simulink model "Backhoe_TiltCyl_PIopt"  (R2018a)
settings: Solver=ode23t  StartTime=0.0  StopTime=30  MaxStep=0.01  RelTol=1e-3  EnableMultiTasking=on
PreLoadFcn:
  | Kp_Final = 19.24;
  | Ki_Final = 0.5024;
  | 
  | Kp_Init = 0.1;
  | Ki_Init = 0.02;
  | 
  | 
  | Kp = Kp_Init;
  | Ki = Ki_Init;
PostLoadFcn:
  | warning off Simulink:Engine:UsingDefaultMaxStepSize
  | warning off Simulink:blocks:MatchingFromNotFound
  | warning off Simulink:Engine:SaveWithParameterizedLinks_Warning
  | warning off Simulink:Engine:SolverMinStepSizeWarnForDAE
model workspace (MAT data in the model file):
  Backhoe_TiltCyl_sdosession = sldodialogs.data.SessionData
  Backhoe_TiltCyl_sdosession.Version = '3.0'
  Backhoe_TiltCyl_sdosession.Data.ModelName = 'Backhoe_TiltCyl_v2'
  Backhoe_TiltCyl_sdosession.Data.GUIOptions.NoPromptClose = 0
  Backhoe_TiltCyl_sdosession.Data.ToolData.PlotManager.Plots.Class = 'sldoplots.TimePlot'
  Backhoe_TiltCyl_sdosession.Data.ToolData.PlotManager.Plots.Sources = {'Bucket_Angle'}
  Backhoe_TiltCyl_sdosession.Data.ToolData.ResponseOptimization.DesignVariables = 'DesignVars'
  Backhoe_TiltCyl_sdosession.Data.ToolData.ResponseOptimization.UncertainVariables = ''
  Backhoe_TiltCyl_sdosession.Data.ToolData.ResponseOptimization.Options = sdo.OptimizeOptions
  Backhoe_TiltCyl_sdosession.Data.ToolData.ResponseOptimization.Options.MethodOptions.Display = 'iter'
  Backhoe_TiltCyl_sdosession.Data.ToolData.ResponseOptimization.Options.MethodOptions.MaxFunEvals = Inf
  Backhoe_TiltCyl_sdosession.Data.ToolData.ResponseOptimization.Options.MethodOptions.MaxIter = 100
  Backhoe_TiltCyl_sdosession.Data.ToolData.ResponseOptimization.Options.MethodOptions.TolFun = 0.001
  Backhoe_TiltCyl_sdosession.Data.ToolData.ResponseOptimization.Options.MethodOptions.TolX = 0.001
  Backhoe_TiltCyl_sdosession.Data.ToolData.ResponseOptimization.Options.MethodOptions.FunValCheck = 'off'
  Backhoe_TiltCyl_sdosession.Data.ToolData.ResponseOptimization.Options.MethodOptions.OutputFcn = []
  Backhoe_TiltCyl_sdosession.Data.ToolData.ResponseOptimization.Options.MethodOptions.PlotFcns = []
  Backhoe_TiltCyl_sdosession.Data.ToolData.ResponseOptimization.Options.MethodOptions.ActiveConstrTol = []
  Backhoe_TiltCyl_sdosession.Data.ToolData.ResponseOptimization.Options.MethodOptions.Algorithm = 'active-set'
  Backhoe_TiltCyl_sdosession.Data.ToolData.ResponseOptimization.Options.MethodOptions.AlwaysHonorConstraints = 'bounds'
  Backhoe_TiltCyl_sdosession.Data.ToolData.ResponseOptimization.Options.MethodOptions.BranchStrategy = []
  Backhoe_TiltCyl_sdosession.Data.ToolData.ResponseOptimization.Options.MethodOptions.DerivativeCheck = 'off'
  Backhoe_TiltCyl_sdosession.Data.ToolData.ResponseOptimization.Options.MethodOptions.Diagnostics = 'off'
  Backhoe_TiltCyl_sdosession.Data.ToolData.ResponseOptimization.Options.MethodOptions.DiffMaxChange = Inf
  Backhoe_TiltCyl_sdosession.Data.ToolData.ResponseOptimization.Options.MethodOptions.DiffMinChange = 0
  Backhoe_TiltCyl_sdosession.Data.ToolData.ResponseOptimization.Options.MethodOptions.FinDiffRelStep = []
  Backhoe_TiltCyl_sdosession.Data.ToolData.ResponseOptimization.Options.MethodOptions.FinDiffType = 'forward'
  Backhoe_TiltCyl_sdosession.Data.ToolData.ResponseOptimization.Options.MethodOptions.GoalsExactAchieve = []
  Backhoe_TiltCyl_sdosession.Data.ToolData.ResponseOptimization.Options.MethodOptions.GradConstr = 'on'
  Backhoe_TiltCyl_sdosession.Data.ToolData.ResponseOptimization.Options.MethodOptions.GradObj = 'on'
  Backhoe_TiltCyl_sdosession.Data.ToolData.ResponseOptimization.Options.MethodOptions.HessFcn = []
  Backhoe_TiltCyl_sdosession.Data.ToolData.ResponseOptimization.Options.MethodOptions.Hessian = []
  Backhoe_TiltCyl_sdosession.Data.ToolData.ResponseOptimization.Options.MethodOptions.HessMult = []
  Backhoe_TiltCyl_sdosession.Data.ToolData.ResponseOptimization.Options.MethodOptions.HessPattern = 'sparse(ones(numberofvariables))'
  Backhoe_TiltCyl_sdosession.Data.ToolData.ResponseOptimization.Options.MethodOptions.HessUpdate = []
  Backhoe_TiltCyl_sdosession.Data.ToolData.ResponseOptimization.Options.MethodOptions.InitialHessType = []
  Backhoe_TiltCyl_sdosession.Data.ToolData.ResponseOptimization.Options.MethodOptions.InitialHessMatrix = []
  Backhoe_TiltCyl_sdosession.Data.ToolData.ResponseOptimization.Options.MethodOptions.InitBarrierParam = 0.1
  Backhoe_TiltCyl_sdosession.Data.ToolData.ResponseOptimization.Options.MethodOptions.InitTrustRegionRadius = 'sqrt(numberofvariables)'
  Backhoe_TiltCyl_sdosession.Data.ToolData.ResponseOptimization.Options.MethodOptions.Jacobian = []
  Backhoe_TiltCyl_sdosession.Data.ToolData.ResponseOptimization.Options.MethodOptions.JacobMult = []
  Backhoe_TiltCyl_sdosession.Data.ToolData.ResponseOptimization.Options.MethodOptions.JacobPattern = []
  Backhoe_TiltCyl_sdosession.Data.ToolData.ResponseOptimization.Options.MethodOptions.LargeScale = 'on'
  Backhoe_TiltCyl_sdosession.Data.ToolData.ResponseOptimization.Options.MethodOptions.LineSearchType = []
  Backhoe_TiltCyl_sdosession.Data.ToolData.ResponseOptimization.Options.MethodOptions.MaxNodes = []
  Backhoe_TiltCyl_sdosession.Data.ToolData.ResponseOptimization.Options.MethodOptions.MaxPCGIter = 'max(1,floor(numberofvariables/2))'
  Backhoe_TiltCyl_sdosession.Data.ToolData.ResponseOptimization.Options.MethodOptions.MaxProjCGIter = '2*(numberofvariables-numberofequalities)'
  Backhoe_TiltCyl_sdosession.Data.ToolData.ResponseOptimization.Options.MethodOptions.MaxRLPIter = []
  Backhoe_TiltCyl_sdosession.Data.ToolData.ResponseOptimization.Options.MethodOptions.MaxSQPIter = '10*max(numberofvariables,numberofinequalities+numberofbounds)'
  Backhoe_TiltCyl_sdosession.Data.ToolData.ResponseOptimization.Options.MethodOptions.MaxTime = []
  Backhoe_TiltCyl_sdosession.Data.ToolData.ResponseOptimization.Options.MethodOptions.MeritFunction = []
  Backhoe_TiltCyl_sdosession.Data.ToolData.ResponseOptimization.Options.MethodOptions.MinAbsMax = []
  Backhoe_TiltCyl_sdosession.Data.ToolData.ResponseOptimization.Options.MethodOptions.NodeDisplayInterval = []
  Backhoe_TiltCyl_sdosession.Data.ToolData.ResponseOptimization.Options.MethodOptions.NodeSearchStrategy = []
  Backhoe_TiltCyl_sdosession.Data.ToolData.ResponseOptimization.Options.MethodOptions.NoStopIfFlatInfeas = 'on'
  Backhoe_TiltCyl_sdosession.Data.ToolData.ResponseOptimization.Options.MethodOptions.ObjectiveLimit = -1e+20
  Backhoe_TiltCyl_sdosession.Data.ToolData.ResponseOptimization.Options.MethodOptions.PhaseOneTotalScaling = 'on'
  Backhoe_TiltCyl_sdosession.Data.ToolData.ResponseOptimization.Options.MethodOptions.Preconditioner = []
  Backhoe_TiltCyl_sdosession.Data.ToolData.ResponseOptimization.Options.MethodOptions.PrecondBandWidth = Inf
  Backhoe_TiltCyl_sdosession.Data.ToolData.ResponseOptimization.Options.MethodOptions.RelLineSrchBnd = 9
  Backhoe_TiltCyl_sdosession.Data.ToolData.ResponseOptimization.Options.MethodOptions.RelLineSrchBndDuration = Inf
  Backhoe_TiltCyl_sdosession.Data.ToolData.ResponseOptimization.Options.MethodOptions.ScaleProblem = 'none'
  Backhoe_TiltCyl_sdosession.Data.ToolData.ResponseOptimization.Options.MethodOptions.Simplex = []
  Backhoe_TiltCyl_sdosession.Data.ToolData.ResponseOptimization.Options.MethodOptions.SubproblemAlgorithm = 'ldl-factorization'
  Backhoe_TiltCyl_sdosession.Data.ToolData.ResponseOptimization.Options.MethodOptions.TolCon = 0.001
  Backhoe_TiltCyl_sdosession.Data.ToolData.ResponseOptimization.Options.MethodOptions.TolConSQP = 1e-06
  Backhoe_TiltCyl_sdosession.Data.ToolData.ResponseOptimization.Options.MethodOptions.TolGradCon = 1e-06
  Backhoe_TiltCyl_sdosession.Data.ToolData.ResponseOptimization.Options.MethodOptions.TolPCG = 0.1
  Backhoe_TiltCyl_sdosession.Data.ToolData.ResponseOptimization.Options.MethodOptions.TolProjCG = 0.01
  Backhoe_TiltCyl_sdosession.Data.ToolData.ResponseOptimization.Options.MethodOptions.TolProjCGAbs = 1e-10
  Backhoe_TiltCyl_sdosession.Data.ToolData.ResponseOptimization.Options.MethodOptions.TolRLPFun = []
  Backhoe_TiltCyl_sdosession.Data.ToolData.ResponseOptimization.Options.MethodOptions.TolXInteger = []
  Backhoe_TiltCyl_sdosession.Data.ToolData.ResponseOptimization.Options.MethodOptions.TypicalX = 'ones(numberofvariables,1)'
  Backhoe_TiltCyl_sdosession.Data.ToolData.ResponseOptimization.Options.MethodOptions.UseParallel = 'never'
  Backhoe_TiltCyl_sdosession.Data.ToolData.ResponseOptimization.Options.OptimizedModel = 'Backhoe_TiltCyl_v2'
  Backhoe_TiltCyl_sdosession.Data.ToolData.ResponseOptimization.GUIOptions.ShowProgress = 1
  Backhoe_TiltCyl_sdosession.Data.ToolData.ResponseOptimization.GUIOptions.UpdatePlots = 1
  Backhoe_TiltCyl_sdosession.Data.ToolData.ResponseOptimization.GUIOptions.UpdateModel = 1
  Backhoe_TiltCyl_sdosession.Data.ToolData.ResponseOptimization.GUIOptions.UpdateDesign = 'overwrite'
  Backhoe_TiltCyl_sdosession.Data.ToolData.ResponseOptimization.GUIOptions.SaveReport = 0
  Backhoe_TiltCyl_sdosession.Data.ToolData.ResponseOptimization.GUIOptions.SaveRequirementValue = 1
  Backhoe_TiltCyl_sdosession.Data.ToolData.ResponseOptimization.DataToPlot = ''
  Backhoe_TiltCyl_sdosession.Data.ToolData.ResponseOptimization.LinOptions = linearize.OldLinoptions
  Backhoe_TiltCyl_sdosession.Data.ToolData.ResponseOptimization.LinOptions.OptimizerType = 'graddescent-elim'
  Backhoe_TiltCyl_sdosession.Data.ToolData.ResponseOptimization.LinOptions.OptimizationOptions.Algorithm = 'active-set'
  Backhoe_TiltCyl_sdosession.Data.ToolData.ResponseOptimization.LinOptions.OptimizationOptions.AlwaysHonorConstraints = 'bounds'
  Backhoe_TiltCyl_sdosession.Data.ToolData.ResponseOptimization.LinOptions.OptimizationOptions.DerivativeCheck = 'off'
  Backhoe_TiltCyl_sdosession.Data.ToolData.ResponseOptimization.LinOptions.OptimizationOptions.Diagnostics = 'off'
  Backhoe_TiltCyl_sdosession.Data.ToolData.ResponseOptimization.LinOptions.OptimizationOptions.DiffMaxChange = Inf
  Backhoe_TiltCyl_sdosession.Data.ToolData.ResponseOptimization.LinOptions.OptimizationOptions.DiffMinChange = 0
  Backhoe_TiltCyl_sdosession.Data.ToolData.ResponseOptimization.LinOptions.OptimizationOptions.Display = 'off'
  Backhoe_TiltCyl_sdosession.Data.ToolData.ResponseOptimization.LinOptions.OptimizationOptions.FinDiffRelStep = []
  Backhoe_TiltCyl_sdosession.Data.ToolData.ResponseOptimization.LinOptions.OptimizationOptions.FinDiffType = 'forward'
  Backhoe_TiltCyl_sdosession.Data.ToolData.ResponseOptimization.LinOptions.OptimizationOptions.FunValCheck = 'off'
  Backhoe_TiltCyl_sdosession.Data.ToolData.ResponseOptimization.LinOptions.OptimizationOptions.GradConstr = 'off'
  Backhoe_TiltCyl_sdosession.Data.ToolData.ResponseOptimization.LinOptions.OptimizationOptions.GradObj = 'off'
  Backhoe_TiltCyl_sdosession.Data.ToolData.ResponseOptimization.LinOptions.OptimizationOptions.HessFcn = []
  Backhoe_TiltCyl_sdosession.Data.ToolData.ResponseOptimization.LinOptions.OptimizationOptions.Hessian = []
  Backhoe_TiltCyl_sdosession.Data.ToolData.ResponseOptimization.LinOptions.OptimizationOptions.HessMult = []
  Backhoe_TiltCyl_sdosession.Data.ToolData.ResponseOptimization.LinOptions.OptimizationOptions.HessPattern = 'sparse(ones(numberOfVariables))'
  Backhoe_TiltCyl_sdosession.Data.ToolData.ResponseOptimization.LinOptions.OptimizationOptions.InitBarrierParam = 0.1
  Backhoe_TiltCyl_sdosession.Data.ToolData.ResponseOptimization.LinOptions.OptimizationOptions.InitTrustRegionRadius = 'sqrt(numberOfVariables)'
  Backhoe_TiltCyl_sdosession.Data.ToolData.ResponseOptimization.LinOptions.OptimizationOptions.MaxFunEvals = 600
  Backhoe_TiltCyl_sdosession.Data.ToolData.ResponseOptimization.LinOptions.OptimizationOptions.MaxIter = 400
  Backhoe_TiltCyl_sdosession.Data.ToolData.ResponseOptimization.LinOptions.OptimizationOptions.MaxPCGIter = 'max(1,floor(numberOfVariables/2))'
  Backhoe_TiltCyl_sdosession.Data.ToolData.ResponseOptimization.LinOptions.OptimizationOptions.MaxProjCGIter = '2*(numberOfVariables-numberOfEqualities)'
  Backhoe_TiltCyl_sdosession.Data.ToolData.ResponseOptimization.LinOptions.OptimizationOptions.MaxSQPIter = '10*max(numberOfVariables,numberOfInequalities+numberOfBounds)'
  Backhoe_TiltCyl_sdosession.Data.ToolData.ResponseOptimization.LinOptions.OptimizationOptions.ObjectiveLimit = -1e+20
  Backhoe_TiltCyl_sdosession.Data.ToolData.ResponseOptimization.LinOptions.OptimizationOptions.OutputFcn = []
  Backhoe_TiltCyl_sdosession.Data.ToolData.ResponseOptimization.LinOptions.OptimizationOptions.PlotFcns = []
  Backhoe_TiltCyl_sdosession.Data.ToolData.ResponseOptimization.LinOptions.OptimizationOptions.PrecondBandWidth = 0
  Backhoe_TiltCyl_sdosession.Data.ToolData.ResponseOptimization.LinOptions.OptimizationOptions.RelLineSrchBnd = []
  Backhoe_TiltCyl_sdosession.Data.ToolData.ResponseOptimization.LinOptions.OptimizationOptions.RelLineSrchBndDuration = 1
  Backhoe_TiltCyl_sdosession.Data.ToolData.ResponseOptimization.LinOptions.OptimizationOptions.ScaleProblem = 'none'
  Backhoe_TiltCyl_sdosession.Data.ToolData.ResponseOptimization.LinOptions.OptimizationOptions.SubproblemAlgorithm = 'ldl-factorization'
  Backhoe_TiltCyl_sdosession.Data.ToolData.ResponseOptimization.LinOptions.OptimizationOptions.TolCon = 1e-06
  Backhoe_TiltCyl_sdosession.Data.ToolData.ResponseOptimization.LinOptions.OptimizationOptions.TolConSQP = 1e-06
  Backhoe_TiltCyl_sdosession.Data.ToolData.ResponseOptimization.LinOptions.OptimizationOptions.TolFun = 1e-06
  Backhoe_TiltCyl_sdosession.Data.ToolData.ResponseOptimization.LinOptions.OptimizationOptions.TolPCG = 0.1
  Backhoe_TiltCyl_sdosession.Data.ToolData.ResponseOptimization.LinOptions.OptimizationOptions.TolProjCG = 0.01
  Backhoe_TiltCyl_sdosession.Data.ToolData.ResponseOptimization.LinOptions.OptimizationOptions.TolProjCGAbs = 1e-10
  Backhoe_TiltCyl_sdosession.Data.ToolData.ResponseOptimization.LinOptions.OptimizationOptions.TolX = 1e-06
  Backhoe_TiltCyl_sdosession.Data.ToolData.ResponseOptimization.LinOptions.OptimizationOptions.TypicalX = 'ones(numberOfVariables,1)'
  Backhoe_TiltCyl_sdosession.Data.ToolData.ResponseOptimization.LinOptions.OptimizationOptions.UseParallel = 0
  Backhoe_TiltCyl_sdosession.Data.ToolData.ResponseOptimization.LinOptions.OptimizationOptions.Jacobian = 'off'
  Backhoe_TiltCyl_sdosession.Data.ToolData.ResponseOptimization.LinOptions.OptimizationOptions.LargeScale = 'off'
  Backhoe_TiltCyl_sdosession.Data.ToolData.ResponseOptimization.LocalRequirements.Requirement = 'SignalTracking'
  Backhoe_TiltCyl_sdosession.Data.ToolData.ResponseOptimization.LocalRequirements.Source = {'Bucket_Angle'}
  Backhoe_TiltCyl_sdosession.Data.ToolData.ResponseOptimization.LocalRequirements.Selected = 1
  Backhoe_TiltCyl_sdosession.Data.ToolData.ResponseOptimization.BlockRequirements = struct([])
  Backhoe_TiltCyl_sdosession.Data.OpenTabs = {'tabResponseOptimization'}
  Backhoe_TiltCyl_sdosession.Data.ToolType = 'ResponseOptimization'
  Backhoe_TiltCyl_sdosession.Data.Workspace.LocalWorkspace.Bucket_Angle = Simulink.SimulationData.Signal
  Backhoe_TiltCyl_sdosession.Data.Workspace.LocalWorkspace.Bucket_Angle.PortType = 'outport'
  Backhoe_TiltCyl_sdosession.Data.Workspace.LocalWorkspace.Bucket_Angle.BlockPath = Simulink.SimulationData.BlockPath
  Backhoe_TiltCyl_sdosession.Data.Workspace.LocalWorkspace.Bucket_Angle.BlockPath.path = {'Backhoe_TiltCyl_v2/Tilt Actuator'}
  Backhoe_TiltCyl_sdosession.Data.Workspace.LocalWorkspace.DesignVars(1) = param.Continuous
  Backhoe_TiltCyl_sdosession.Data.Workspace.LocalWorkspace.DesignVars(1).Minimum_ = 0
  Backhoe_TiltCyl_sdosession.Data.Workspace.LocalWorkspace.DesignVars(1).Scale_ = 0.25
  Backhoe_TiltCyl_sdosession.Data.Workspace.LocalWorkspace.DesignVars(1).Size_ = [1 1]
  Backhoe_TiltCyl_sdosession.Data.Workspace.LocalWorkspace.DesignVars(1).Value_ = 0.2
  Backhoe_TiltCyl_sdosession.Data.Workspace.LocalWorkspace.DesignVars(1).pID = paramid.Variable
  Backhoe_TiltCyl_sdosession.Data.Workspace.LocalWorkspace.DesignVars(1).pID.Name = 'Ki'
  Backhoe_TiltCyl_sdosession.Data.Workspace.LocalWorkspace.DesignVars(2) = param.Continuous
  Backhoe_TiltCyl_sdosession.Data.Workspace.LocalWorkspace.DesignVars(2).Minimum_ = 0
  Backhoe_TiltCyl_sdosession.Data.Workspace.LocalWorkspace.DesignVars(2).Scale_ = 16
  Backhoe_TiltCyl_sdosession.Data.Workspace.LocalWorkspace.DesignVars(2).Size_ = [1 1]
  Backhoe_TiltCyl_sdosession.Data.Workspace.LocalWorkspace.DesignVars(2).Value_ = 10
  Backhoe_TiltCyl_sdosession.Data.Workspace.LocalWorkspace.DesignVars(2).pID = paramid.Variable
  Backhoe_TiltCyl_sdosession.Data.Workspace.LocalWorkspace.DesignVars(2).pID.Name = 'Kp'
  Backhoe_TiltCyl_sdosession.Data.Workspace.LocalWorkspace.SignalTracking = sdo.requirements.SignalTracking
  Backhoe_TiltCyl_sdosession.Data.Workspace.LocalWorkspace.SignalTracking.any.ReferenceSignal = timeseries
  Backhoe_TiltCyl_sdosession.Data.Workspace.LocalWorkspace.SignalTracking.any.ReferenceSignal.Name = 'unnamed'
  Backhoe_TiltCyl_sdosession.Data.Workspace.LocalWorkspace.SignalTracking.any.ReferenceSignal.DataInfo = tsdata.datametadata
  Backhoe_TiltCyl_sdosession.Data.Workspace.LocalWorkspace.SignalTracking.any.ReferenceSignal.DataInfo.Interpolation = tsdata.interpolation
  Backhoe_TiltCyl_sdosession.Data.Workspace.LocalWorkspace.SignalTracking.any.ReferenceSignal.DataInfo.Interpolation.Fhandle : function handle (value not decoded)
  Backhoe_TiltCyl_sdosession.Data.Workspace.LocalWorkspace.SignalTracking.any.ReferenceSignal.DataInfo.Interpolation.Name = 'linear'
  Backhoe_TiltCyl_sdosession.Data.Workspace.LocalWorkspace.SignalTracking.any.ReferenceSignal.TimeInfo = tsdata.timemetadata
  Backhoe_TiltCyl_sdosession.Data.Workspace.LocalWorkspace.SignalTracking.any.ReferenceSignal.TimeInfo.Length = 6
  Backhoe_TiltCyl_sdosession.Data.Workspace.LocalWorkspace.SignalTracking.any.ReferenceSignal.TimeInfo.DuplicateTimes = 0
  Backhoe_TiltCyl_sdosession.Data.Workspace.LocalWorkspace.SignalTracking.any.ReferenceSignal.TimeInfo.Time_ = [0; 7; 11; 24; 28.5; 30]
  Backhoe_TiltCyl_sdosession.Data.Workspace.LocalWorkspace.SignalTracking.any.ReferenceSignal.TimeInfo.Initialized = 1
  Backhoe_TiltCyl_sdosession.Data.Workspace.LocalWorkspace.SignalTracking.any.ReferenceSignal.QualityInfo = tsdata.qualmetadata
  Backhoe_TiltCyl_sdosession.Data.Workspace.LocalWorkspace.SignalTracking.any.ReferenceSignal.Data_ = [0; 0; -90; -90; 0; 0]
  Backhoe_TiltCyl_sdosession.Data.Workspace.LocalWorkspace.SignalTracking.any.ReferenceSignal.Version = 10.1
  Backhoe_TiltCyl_sdosession.Data.Workspace.LocalWorkspace.SignalTracking.any.Weights = [1; 1; 1; 1; 1; 1]
  Backhoe_TiltCyl_sdosession.Data.Workspace.LocalWorkspace.SignalTracking.any.Type = '=='
  Backhoe_TiltCyl_sdosession.Data.Workspace.LocalWorkspace.SignalTracking.any.Method = 'SSE'
  Backhoe_TiltCyl_sdosession.Data.Workspace.LocalWorkspace.SignalTracking.any.InterpolationTimes = 'Reference only'
  Backhoe_TiltCyl_sdosession.Data.Workspace.LocalWorkspace.SignalTracking.any.Normalize = 'on'
  Backhoe_TiltCyl_sdosession.Data.Workspace.LocalWorkspace.SignalTracking.any.RobustCost = 'off'
  Backhoe_TiltCyl_sdosession.Data.Workspace.LocalWorkspace.SignalTracking.any.RelTol = 0
  Backhoe_TiltCyl_sdosession.Data.Workspace.LocalWorkspace.SignalTracking.any.AbsTol = 0
  Backhoe_TiltCyl_sdosession.Data.Workspace.LocalWorkspace.SignalTracking.any.Name = ''
  Backhoe_TiltCyl_sdosession.Data.Workspace.LocalWorkspace.SignalTracking.any.Description = ''
  Backhoe_TiltCyl_sdosession.Data.Workspace.HiddenWorkspace = []
  cylinderGray = [0.6 0.6 0.6]
  darkOrange = [0.8 0.5 0]
  glassBlue = [0.2 0.2 1]
  gray = [0.3 0.3 0.3]
  orange = [0.8 0.65 0]
  pistonGray = [0.4 0.4 0.4]
  rhoGlass = 2500
  rhoRubber = 1500
  rhoSteel = 7800
  tireBlack = [0.1 0.1 0.1]
  wheelGray = [0.6 0.6 0.6]
  yellow = [0.8 0.8 0]
undefined symbols (not defined in the file or in its folder): BH_Param, sigbuilder_block, X, Y, Z
libraries: sm_lib x54, fl_lib x16, Backhoe_Lib x15, nesl_utility x7, sh_lib x5
(part 1 of 2)
Description:
  | Copyright 2014-2018 The MathWorks, Inc.
settings Model: Creator=smiller  LastModifiedBy=smiller
settings DataIOCC: SaveFormat=Array
settings OptimizationCC: ExpressionDepthLimit=2147483647  LifeSpan=inf
settings DebuggingCC: UnderspecifiedInitializationDetection=Classic  MergeDetectMultiDrivingBlocksExec=none  SolverPrmCheckMsg=warning  AllowSymbolicDim=off  StateNameClashWarn=warning  SFUnexpectedBacktrackingDiag=warning  SFNoUnconditionalDefaultTransitionDiag=warning  SFExecutionAtInitializationDiag=none
settings HardwareCC: ProdBitPerPointer=32  ProdBitPerSizeT=32  ProdBitPerPtrDiffT=32  ProdLargestAtomicFloat=None  ProdIntDivRoundTo=Undefined  ProdEndianess=Unspecified  ProdWordSize=32  ProdHWDeviceType=32-bit Generic
settings ModelReferenceCC: PropagateSignalLabelsOutOfModel=off
settings CodeAppCC: StateflowObjectComments=on
settings GRTTargetCC: TargetLangStandard=C89/C90 (ANSI)  GeneratePreprocessorConditionals=Disable all
settings ConfigComp: CovMetricSettings=dw  CovHtmlReporting=on  CovSaveCumulativeToWorkspaceVar=on  CovSaveSingleToWorkspaceVar=on  CovExternalEMLEnable=off  CovSFcnEnable=off
settings SimscapeCC: SimscapeNormalizeSystem=off  SimscapeLogType=all  SimscapeLogName=simlog_Backhoe_TiltCyl_PIopt  SimscapeLogDataHistory=80000
settings ConfigurationSet: Description=SimMechanics 2G
settings ExplorerConfigSet: InternalSimMechanicsExplorerSettings="<ExplorerConfiguration><canonicalview>default</canonicalview><TilePanel><TileInfo><Tiles Columns=\"1\" Count=\"1\" Rows=\"1\"><Column Left=\"2\" Weight=\"1\"/><Column Left=\"384\"/><Row Top=\"2\" Weight=\"1\"/><Row Top=\"405\"/><Tile Height=\"1\" Width=\"1\" X=\"0\" Y=\"0\"/></Tiles></TileInfo><SceneInfo><SceneViewer><BGColor><R>0.60000002384185791</R><G>0.60000002384185791</G><B>0.60000002384185791</B></BGColor><Camera><Position><X>2.6903005851409905</X><Y>-1.8683919492819583</Y><Z>-11.77401628900504</Z></Position><Center><X>2.5402467250823975</X><Y>-1.1818122863769531</Y><Z>0</Z></Center><Up><X>0.72882195520801829</X><Y>-0.68293959457603104</Y><Z>0.049112806548679153</Z></Up><Left>-4.5740998506546022</Left><Right>4.5740998506546022</Right><Bottom>-4.7455819129943846</Bottom><Top>4.7455819129943846</Top></Camera></SceneViewer></SceneInfo></TilePanel></ExplorerConfiguration>"

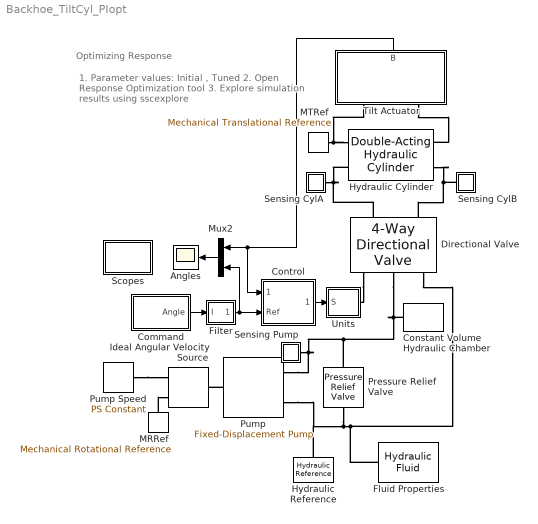
== system Backhoe_TiltCyl_PIopt ==
  note: 1. Parameter values: Initial , Tuned
      | 2. Open Response Optimization tool
      | 3. Explore simulation results
      | using sscexplore
  note: Optimizing Response
  Angles : Scope
  Command : Subsystem  Tag=STV Subsys  LoadFcn=sigbuilder_block('load');  StartFcn=sigbuilder_block('start');  StopFcn=sigbuilder_block('stop');  ClipboardFcn=sigbuilder_block('clipboard');  mask(Sigbuilder block){tuvar=[0:10]}
      mask help: Simulink:masks:SigbuilderBlock_MD
      mask init:
      | if ~strcmp(get_param(bdroot(gcbh),'SimulationStatus'),'stopped') tuvar = sigbuilder_block('maskInit'); end
      settings: CopyFcn=sigbuilder_block('copy');  DeleteFcn=sigbuilder_block('delete');  ModelCloseFcn=sigbuilder_block('modelClose');  PreSaveFcn=sigbuilder_block('preSave');  PauseFcn=sigbuilder_block('pause');  ContinueFcn=sigbuilder_block('continue');  NameChangeFcn=sigbuilder_block('namechange');  OpenFcn=sigbuilder_block('open',[5.58621 9.31034 624.414 409.034 ]);  CloseFcn=sigbuilder_block('close');
      mask Display: plot(0, 0, 100, 100,[2, 2, 32, 32, 2], [68, 8, 8, 68, 68],[32, 2], [38, 38], [32, 19, 2],[53, 60, 44], [32, 17, 17, 2],[16, 16, 31, 31]);txt = getActiveGroup(gcbh);text(2, 100, txt,'verticalAlignment', 'top');
  Constant Volume Hydraulic Chamber : fl_lib/Hydraulic/Hydraulic Elements/Constant Volume Hydraulic Chamber  ch_sp=1  wall_type=1  ch_volume=1e-4 m^3  d_in=1e-2 m  length=1 m  pr_r_coef=1.2e-12 m/Pa  time_const=0.01 s  k_sh=1.4  pressure_specify=off  pressure_priority=High  pressure=0 Pa  pressure_nominal_specify=off  pressure_nominal_unit=Pa  pressure_nominal_value=1  diameter_incr_specify=off  diameter_incr_priority=High  diameter_incr=0 m  diameter_incr_nominal_specify=off  diameter_incr_nominal_unit=m  diameter_incr_nominal_value=1  flow_rate_specify=off  flow_rate_priority=None  flow_rate=0.001 m^3/s  flow_rate_nominal_specify=off  flow_rate_nominal_unit=m^3/s  flow_rate_nominal_value=1
      settings: SourceProductName=Simscape  SourceProductBaseCode=SS
  Control : Subsystem  mask(PID Controller){upperLim=10, lowerLim=-120, Kp=Kp, Ki=Ki, Kd=0.2, N=100}
      mask prompts: upperLim "Upper Limit [deg]"; lowerLim "Lower Limit [deg]"
      mask help: This block takes in a reference angle and measured angle, and uses a PID Controller with saturation to give a control command.
  Directional Valve : sh_lib/Valves/Directional Valves/4-Way Directional Valve  Tag=Factory Generic  area_spec=1  mdl_type_identical=1  mdl_type_different=1  opening_max=BH_Param.Tilt_Actuator.Valve.Max_Opening m  area_max=BH_Param.Tilt_Actuator.Valve.Max_Area mm^2  opening_max_P_A=0.005 m  area_max_P_A=0.5e-4 m^2  opening_max_P_B=0.005 m  area_max_P_B=0.5e-4 m^2  opening_max_A_T=0.005 m  area_max_A_T=0.5e-4 m^2  opening_max_B_T=0.005 m  area_max_B_T=0.5e-4 m^2  opening_area_tab="[  -0.002 0 0.005 0.015 ] m"  area_tab="[  1e-12 4e-12 1e-05 1.02e-05 ] m^2"  opening_flow_rate_tab="[  -0.002 0 0.005 0.015 ] m"  pressure_tab="[  -5e+06 -2e+06 2e+06 5e+06 ] Pa"  flow_rate_tab="[  -1e-12 -6e-14 6e+12 1e+11 ; -8e-08 -4e-08 4e+06 8e+06 ; -0.0025 -0.00103 0.001 0.0024 ; -0.00258 -0.001032 0.00106 0.00247 ; ] m^3/s"  opening_area_tab_P_A=[-0.002, 0.0, 0.002, 0.005, 0.015] m  area_tab_P_A=[1.0e-9, 2.0352e-7, 4.0736e-5, 0.00011438, 0.00034356] m^2  opening_flow_rate_tab_P_A=[-0.002, 0.0, 0.002, 0.005, 0.015] m  pressure_tab_P_A=[-10000000.0, -5000000.0, -2000000.0, 2000000.0, 5000000.0, 10000000.0] Pa  flow_rate_tab_P_A=[-1.0e-7, -7.0711e-8, -4.4721e-8, 4.4721e-8, 7.0711e-8, 1.0e-7; -2.0352e-5, -1.4391e-5, -9.1017e-6, 9.1017e-6, 1.4391e-5, 2.0352e-5; -0.0040736, -0.0028805, -0.0018218, 0.0018218, 0.0028805, 0.0040736; -0.011438, -0.0080879, -0.0051152, 0.0051152, 0.0080879, 0.011438; -0.034356, -0.024293, -0.015364, 0.015364, 0.024293, 0.034356] m^3/s  opening_area_tab_P_B=[-0.002, 0.0, 0.002, 0.005, 0.015] m  area_tab_P_B=[1.0e-9, 2.0352e-7, 4.0736e-5, 0.00011438, 0.00034356] m^2  opening_flow_rate_tab_P_B=[-0.002, 0.0, 0.002, 0.005, 0.015] m  pressure_tab_P_B=[-10000000.0, -5000000.0, -2000000.0, 2000000.0, 5000000.0, 10000000.0] Pa  flow_rate_tab_P_B=[-1.0e-7, -7.0711e-8, -4.4721e-8, 4.4721e-8, 7.0711e-8, 1.0e-7; -2.0352e-5, -1.4391e-5, -9.1017e-6, 9.1017e-6, 1.4391e-5, 2.0352e-5; -0.0040736, -0.0028805, -0.0018218, 0.0018218, 0.0028805, 0.0040736; -0.011438, -0.0080879, -0.0051152, 0.0051152, 0.0080879, 0.011438; -0.034356, -0.024293, -0.015364, 0.015364, 0.024293, 0.034356] m^3/s  opening_area_tab_A_T=[-0.002, 0.0, 0.002, 0.005, 0.015] m  area_tab_A_T=[1.0e-9, 2.0352e-7, 4.0736e-5, 0.00011438, 0.00034356] m^2  opening_flow_rate_tab_A_T=[-0.002, 0.0, 0.002, 0.005, 0.015] m  pressure_tab_A_T=[-10000000.0, -5000000.0, -2000000.0, 2000000.0, 5000000.0, 10000000.0] Pa  flow_rate_tab_A_T=[-1.0e-7, -7.0711e-8, -4.4721e-8, 4.4721e-8, 7.0711e-8, 1.0e-7; -2.0352e-5, -1.4391e-5, -9.1017e-6, 9.1017e-6, 1.4391e-5, 2.0352e-5; -0.0040736, -0.0028805, -0.0018218, 0.0018218, 0.0028805, 0.0040736; -0.011438, -0.0080879, -0.0051152, 0.0051152, 0.0080879, 0.011438; -0.034356, -0.024293, -0.015364, 0.015364, 0.024293, 0.034356] m^3/s  opening_area_tab_B_T=[-0.002, 0.0, 0.002, 0.005, 0.015] m  area_tab_B_T=[1.0e-9, 2.0352e-7, 4.0736e-5, 0.00011438, 0.00034356] m^2  opening_flow_rate_tab_B_T=[-0.002, 0.0, 0.002, 0.005, 0.015] m  pressure_tab_B_T=[-10000000.0, -5000000.0, -2000000.0, 2000000.0, 5000000.0, 10000000.0] Pa  flow_rate_tab_B_T=[-1.0e-7, -7.0711e-8, -4.4721e-8, 4.4721e-8, 7.0711e-8, 1.0e-7; -2.0352e-5, -1.4391e-5, -9.1017e-6, 9.1017e-6, 1.4391e-5, 2.0352e-5; -0.0040736, -0.0028805, -0.0018218, 0.0018218, 0.0028805, 0.0040736; -0.011438, -0.0080879, -0.0051152, 0.0051152, 0.0080879, 0.011438; -0.034356, -0.024293, -0.015364, 0.015364, 0.024293, 0.034356] m^3/s  interp_method_identical=1  interp_method_different=1  extrap_method_identical=1  extrap_method_different=1  C_d=0.7  x_0_P_A=-1e-4 m  x_0_P_B=-1e-4 m  x_0_A_T=-1e-4 m  x_0_B_T=-1e-4 m  A_leak=1e-12 m^2  lam_spec=2  B_lam=0.999  Re_cr=12
      settings: SourceProductName=Simscape Fluids  SourceProductBaseCode=SH
  Filter : Subsystem  mask{b=1e-1, x_initial=0}
      mask prompts: b "Filter time constant"; x_initial "Initial Output"
  Fluid Properties : sh_lib/Hydraulic Utilities/Hydraulic Fluid  DataSource=1  SelFluid=9  SysTemp=50  TrapAir=0.004  ViscDerFactor=1  range_error=2
      settings: SourceProductName=Simscape Fluids
  Hydraulic Reference : fl_lib/Hydraulic/Hydraulic Elements/Hydraulic Reference
      settings: SourceProductName=Simscape
  Hydraulic Cylinder : sh_lib/Hydraulic Cylinders/Double-Acting Hydraulic Cylinder  Tag=Factory Generic  area_A=BH_Param.Tilt_Actuator.Cylinder.Area_A m^2  area_B=BH_Param.Tilt_Actuator.Cylinder.Area_B m^2  stroke=BH_Param.Tilt_Actuator.Cylinder.Stroke m  init_pos=BH_Param.Tilt_Actuator.Cylinder.x0 m  dead_vol_A=BH_Param.Tilt_Actuator.Cylinder.DeadVol_A m^3  dead_vol_B=BH_Param.Tilt_Actuator.Cylinder.DeadVol_B m^3  init_pressure_A=1.45e7 Pa  init_pressure_B=1.31e7 Pa  k_sh=1.4  stiff=1e+06 N/m  D=150 N/(m/s)  hardstop_model=3  transition=0.1 mm  or=2
      settings: SourceProductName=Simscape Fluids  SourceProductBaseCode=SH
  Ideal Angular Velocity Source : fl_lib/Mechanical/Mechanical Sources/Ideal Angular Velocity Source
  MRRef : fl_lib/Mechanical/Rotational Elements/Mechanical Rotational Reference
  MTRef : fl_lib/Mechanical/Translational Elements/Mechanical Translational Reference  Tag=Factory Generic
  Mux2 : Mux  Inputs=2
  Pressure Relief Valve : sh_lib/Valves/Pressure Control Valves/Pressure Relief Valve  valve_area_spec=1  p_diff_TLU=[30.15e5 : 15e3 : 31.35e5] Pa  area_TLU=[1 : 1 : 9] .* 1e-5 m^2  area_max=BH_Param.Hydraulic.PRV.Max_Area m^2  pres_set=BH_Param.Hydraulic.PRV.Pressure_Set Pa  reg_range=BH_Param.Hydraulic.PRV.Pressure_Rng Pa  C_d=BH_Param.Hydraulic.PRV.Flow_Disch_Coeff  A_leak=BH_Param.Hydraulic.PRV.Leakage_Area m^2  lam_spec=2  B_lam=0.999  Re_cr=BH_Param.Hydraulic.PRV.Re_Critical  dynamic=0  tau=0.1 s  area_init=1e-12 m^2
      settings: SourceProductName=Simscape Fluids  SourceProductBaseCode=SH
  Pump : sh_lib/Pumps and Motors/Fixed-Displacement Pump  D=BH_Param.Hydraulic.Pump.Displacement m^3/rad  loss_spec=1  w_nominal=BH_Param.Hydraulic.Pump.Nominal_Ang_Vel rad/s  pr_nominal=BH_Param.Hydraulic.Pump.Nominal_Pressure Pa  visc_nominal=BH_Param.Hydraulic.Pump.Nominal_Kin_Visc cSt  dens_nominal=900 kg/m^3  efficiency_vol=BH_Param.Hydraulic.Pump.Vol_Eff  no_load_torque=0 N*m  torque_pressure_coeff=1*(BH_Param.Hydraulic.Pump.Displacement)*((BH_Param.Hydraulic.Pump.Vol_Eff)/(BH_Param.Hydraulic.Pump.Total_Eff)-1 ) N*m/Pa  p_diff_eff_TLU=[100000.0, 1000000.0, 2000000.0] Pa  omega_eff_TLU=[25.0, 50.0, 100.0, 200.0, 300.0, 400.0] rad/s  vol_eff_TLU=[0.816, 0.908, 0.954, 0.977, 0.981, 0.984; 0.325, 0.663, 0.831, 0.916, 0.925, 0.946; 0.137, 0.568, 0.78, 0.892, 0.893, 0.91]  mech_eff_TLU=[0.996, 0.996, 0.996, 0.996, 0.996, 0.996; 0.988, 0.989, 0.989, 0.989, 0.989, 0.99; 0.981, 0.981, 0.982, 0.982, 0.983, 0.984]  p_diff_loss_TLU=[100000.0, 1000000.0, 2000000.0] Pa  omega_loss_TLU=[25.0, 50.0, 100.0, 200.0, 300.0, 400.0] rad/s  vol_loss_TLU=[0.023, 0.023, 0.023, 0.023, 0.0285, 0.032; 0.0844, 0.0842, 0.0845, 0.084, 0.1125, 0.108; 0.1079, 0.108, 0.11, 0.108, 0.1605, 0.18] * 1e-3 m^3/s  mech_loss_TLU=[0.002, 0.002, 0.002, 0.002, 0.002, 0.002; 0.0607, 0.0556, 0.0556, 0.0556, 0.0556, 0.0505; 0.1937, 0.1937, 0.1833, 0.1833, 0.1729, 0.1626] N*m  pressure_threshold=1e5 Pa  omega_threshold=10 rad/s  quadrant_check=0  pressure_check=0  min_valid_pressure=0 Pa  vol_eff_min=1e-3  vol_eff_max=1  mech_eff_min=1e-3  mech_eff_max=1
      settings: SourceProductName=Simscape Fluids  SourceProductBaseCode=SH
  Pump Speed : fl_lib/Physical Signals/Sources/PS Constant  constant=188
  Scopes : Subsystem
  Sensing CylA : Subsystem
      mask Display: disp('S')
  Sensing CylB : Subsystem
      mask Display: disp('S')
  Sensing Pump : Subsystem
      mask Display: disp('S')
  Tilt Actuator : Subsystem
      mask Display:
      | image(imread('Backhoe_Tilt_Actuator_IMAGE.jpg'));
      | port_label('lconn',1,'C');
      | port_label('lconn',2,'R');
      | port_label('output',1,'B');
  Units : Subsystem
  wires:
  Command/1(Angle) -> Filter/1(I)
  Tilt Actuator/1(B) -> Mux2/1, Control/1(Meas)
  Control/1(Cmd) -> Units/1(S)
  Mux2/1 -> Angles/1
  Filter/1(O) -> Mux2/2, Control/2(Ref)
  connections:
  Directional Valve/RConn2 -- Pump/RConn1 -- Sensing Pump/LConn1 -- Pressure Relief Valve/LConn1 -- Constant Volume Hydraulic Chamber/LConn1
  Directional Valve/RConn3 -- Fluid Properties/RConn1 -- Pump/RConn2 -- Hydraulic Reference/LConn1 -- Pressure Relief Valve/RConn1
  MRRef/LConn1 -- Ideal Angular Velocity Source/RConn2
  Pump/LConn1 -- Ideal Angular Velocity Source/LConn1
  Pump Speed/RConn1 -- Ideal Angular Velocity Source/RConn1
  Sensing CylB/LConn1 -- Directional Valve/LConn2 -- Hydraulic Cylinder/RConn2
  Hydraulic Cylinder/LConn1 -- Tilt Actuator/LConn1 -- MTRef/LConn1
  Hydraulic Cylinder/LConn2 -- Directional Valve/LConn1 -- Sensing CylA/LConn1
  Tilt Actuator/LConn2 -- Hydraulic Cylinder/RConn1
  Directional Valve/RConn1 -- Units/RConn1

== system Backhoe_TiltCyl_PIopt/Command ==
  Demux : Demux  Tag=STV Demux  Outputs=1
  FromWs : FromWorkspace  Tag=STV FromWs  VariableName=tuvar  SampleTime=0  OutputAfterFinalValue=Holding final value
      SigBuilderData=|
      | common.afterFinalStr = 'Hold final value'
      | common.sampleTime = '0'
      | dataSet.timeRange = [0 60]
      | dataSet.name = 'Ref'
      | sbobj.Groups.Name = 'Ref'
      | sbobj.Groups.Signals.Name = 'Angle'
      | sbobj.Groups.Signals.XData = [0 7 11 24 28.5 40 42 51.5 53.5 60]
      | sbobj.Groups.Signals.YData = [0 0 -90 -90 0 0 -110 -110 0 0]
      | sbobj.Groups.TimeRange = [0 60]
  Angle : Outport  Tag=STV Outport
  wires:
  Demux/1 -> Angle/1
  FromWs/1 -> Demux/1

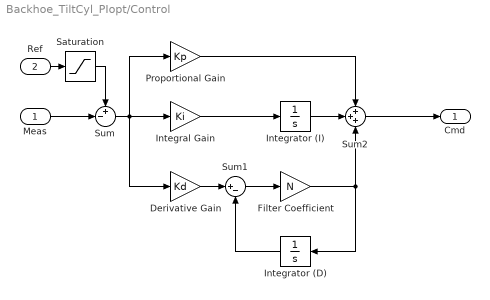
== system Backhoe_TiltCyl_PIopt/Control ==
  Meas : Inport
  Ref : Inport  Port=2
  Derivative Gain : Gain  Gain=Kd
  Filter Coefficient : Gain  Gain=N
  Integral Gain : Gain  Gain=Ki
  Integrator (D) : Integrator
  Integrator (I) : Integrator
  Proportional Gain : Gain  Gain=Kp
  Saturation : Saturate  UpperLimit=upperLim  LowerLimit=lowerLim
  Sum : Sum  Inputs=+-|
  Sum1 : Sum  Inputs=|+-
  Sum2 : Sum  Inputs=+++
  Cmd : Outport
  wires:
  Saturation/1 -> Sum/1
  Meas/1 -> Sum/2
  Ref/1 -> Saturation/1
  Sum/1 -> Integral Gain/1, Proportional Gain/1, Derivative Gain/1
  Integrator (I)/1 -> Sum2/2
  Integrator (D)/1 -> Sum1/2
  Filter Coefficient/1 -> Integrator (D)/1, Sum2/3
  Sum1/1 -> Filter Coefficient/1
  Derivative Gain/1 -> Sum1/1
  Integral Gain/1 -> Integrator (I)/1
  Proportional Gain/1 -> Sum2/1
  Sum2/1 -> Cmd/1

== system Backhoe_TiltCyl_PIopt/Filter ==
  I : Inport
  Gain : Gain  Gain=1/b
  Integrator : Integrator  InitialCondition=x_initial
  Sum : Sum  Inputs=|+-
  O : Outport
  wires:
  Gain/1 -> Integrator/1
  Integrator/1 -> O/1, Sum/2
  I/1 -> Sum/1
  Sum/1 -> Gain/1

== system Backhoe_TiltCyl_PIopt/Scopes ==
  Cylinder Pressures : Scope
  Force : Scope
  Mux : Mux  Inputs=2
  wires:
  [Tilt_PB] -> Mux/2
  [Tilt_PA] -> Mux/1
  Mux/1 -> Cylinder Pressures/1
  [Tilt_Act_F] -> Force/1  "Force"

== system Backhoe_TiltCyl_PIopt/Sensing CylA ==
  Hydraulic Pressure Sensor : fl_lib/Hydraulic/Hydraulic Sensors/Hydraulic Pressure Sensor
      settings: SourceProductName=Simscape
  Hydraulic Reference1 : fl_lib/Hydraulic/Hydraulic Elements/Hydraulic Reference
      settings: SourceProductName=Simscape
  PS-Simulink Converter1 : nesl_utility/PS-Simulink Converter  PhysicalDomain=network_engine_domain  SubClassName=ps_output  LeftPortType=input  RightPortType=output  PseudoPeriodic=off  Frequencies=[]  Unit=Pa  AffineConversion=off
  A : PMIOPort  Side=Left
  tag scope: Tilt_PA=global
  wires:
  PS-Simulink Converter1/1 -> [Tilt_PA]
  connections:
  PS-Simulink Converter1/LConn1 -- Hydraulic Pressure Sensor/RConn2
  Hydraulic Reference1/LConn1 -- Hydraulic Pressure Sensor/RConn1
  Hydraulic Pressure Sensor/LConn1 -- A/RConn1

== system Backhoe_TiltCyl_PIopt/Sensing CylB ==
  Hydraulic Pressure Sensor : fl_lib/Hydraulic/Hydraulic Sensors/Hydraulic Pressure Sensor
      settings: SourceProductName=Simscape
  Hydraulic Reference1 : fl_lib/Hydraulic/Hydraulic Elements/Hydraulic Reference
      settings: SourceProductName=Simscape
  PS-Simulink Converter1 : nesl_utility/PS-Simulink Converter  PhysicalDomain=network_engine_domain  SubClassName=ps_output  LeftPortType=input  RightPortType=output  PseudoPeriodic=off  Frequencies=[]  Unit=Pa  AffineConversion=off
  A : PMIOPort  Side=Left
  tag scope: Tilt_PB=global
  wires:
  PS-Simulink Converter1/1 -> [Tilt_PB]
  connections:
  Hydraulic Pressure Sensor/LConn1 -- A/RConn1
  Hydraulic Reference1/LConn1 -- Hydraulic Pressure Sensor/RConn1
  PS-Simulink Converter1/LConn1 -- Hydraulic Pressure Sensor/RConn2

== system Backhoe_TiltCyl_PIopt/Sensing Pump ==
  Hydraulic Pressure Sensor : fl_lib/Hydraulic/Hydraulic Sensors/Hydraulic Pressure Sensor
      settings: SourceProductName=Simscape
  Hydraulic Reference1 : fl_lib/Hydraulic/Hydraulic Elements/Hydraulic Reference
      settings: SourceProductName=Simscape
  PS-Simulink Converter1 : nesl_utility/PS-Simulink Converter  PhysicalDomain=network_engine_domain  SubClassName=ps_output  LeftPortType=input  RightPortType=output  PseudoPeriodic=off  Frequencies=[]  Unit=1  AffineConversion=off
  A : PMIOPort  Side=Left
  tag scope: Lift_PP=global
  wires:
  PS-Simulink Converter1/1 -> [Lift_PP]
  connections:
  PS-Simulink Converter1/LConn1 -- Hydraulic Pressure Sensor/RConn2
  Hydraulic Reference1/LConn1 -- Hydraulic Pressure Sensor/RConn1
  Hydraulic Pressure Sensor/LConn1 -- A/RConn1

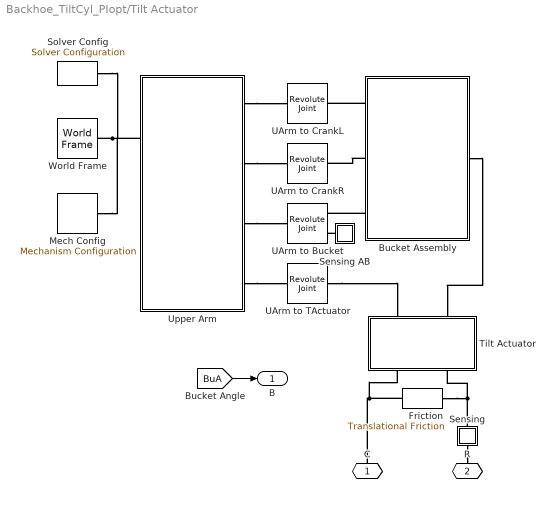
== system Backhoe_TiltCyl_PIopt/Tilt Actuator ==
  Bucket Assembly : Subsystem
      mask Display:
      | image(imread('Backhoe_Arm_Bucket_Asy_IMAGE.JPG'));
      | port_label('lconn',1,'UAL');
      | port_label('lconn',2,'UAR');
      | port_label('lconn',3,'UA');
      | port_label('rconn',1,'TAct');
  Friction : fl_lib/Mechanical/Translational Elements/Translational Friction  brkwy_frc=BH_Param.Tilt_Actuator.Friction.Breakaway N  brkwy_vel=0.060623 m/s  Col_frc=BH_Param.Tilt_Actuator.Friction.Coulomb N  visc_coef=BH_Param.Tilt_Actuator.Friction.Viscous N/(m/s)  v_specify=off  v_priority=High  v=0 m/s  v_nominal_specify=off  v_nominal_unit=m/s  v_nominal_value=1  f_specify=off  f_priority=High  f=0 N  f_nominal_specify=off  f_nominal_unit=N  f_nominal_value=1
      settings: SourceProductName=Simscape  SourceProductBaseCode=SS
  Mech Config : sm_lib/Utilities/Mechanism Configuration  UniformGravity=Constant  GravityVector=[0 -9.81 0]  GravityUnits=m/s^2  LinearizationDelta=0.001
  Sensing : Subsystem
      mask Display: disp('S')
  Sensing AB : Subsystem
      mask Display: disp('S')
  Solver Config : nesl_utility/Solver Configuration  PhysicalDomain=network_engine_domain  SubClassName=solver  LeftPortType=input  RightPortType=generic  Tones=[]  Harmonics=[]  SimulateNoise=off  Profile=off  UseLocalSampling=off  EnableSwitchedLinearOptims=on  FrequencyDomain=off  UseCCode=off  RelTol=0.001  AbsTol=1e-06  MinStep=1e-09  ToWorkspace=off  RevertToSquareIcSolve=off  NumHomotopyIterations=100  PhasorMode=off  PhasorModeNumHarmonics=1  DoDC=off  ResidualTolerance=1e-9  UseLocalSolver=off  LocalSolverChoice=NE_BACKWARD_EULER_ADVANCER  LocalSolverSampleTime=.001  DoFixedCost=off  MaxNonlinIter=3  MaxModeIter=2  LinearAlgebra=Sparse  EquationFormulation=NE_TIME_EF  DelaysMemoryBudget=1024  AutomaticFiltering=on  FilteringTimeConstant=0.001
  Tilt Actuator : Subsystem  mask(Hydraulic Actuator){Lcyl=1.9, Rcyl=0.2, Lpist=1.9, Rpist=0.12, Lbase=0.65, Wbase=0.425, Rbp=0.075, Lbp=0.8, Whead=0.35, Lhead=0.65, Rhp=0.075, Lhp=0.9, circlePoints=25, cylColor=BH_Param.Colors.cylinderGray, rhoCyl=BH_Param.Densities.rhoSteel, pistColor=BH_Param.Colors.pistonGray, rhoPist=BH_Param.Densities.rhoSteel, connColor=BH_Param.Colors.gray, rhoConn=BH_Param.Densities.rhoSteel}
      mask prompts: Lcyl "Lcyl [m]"; Rcyl "Rcyl [m]"; Lpist "Lpist [m]"; Rpist "Rpist [m]"; Lbase "Lbase [m]"; Wbase "Wbase [m]"; Rbp "Rbp [m]"; Lbp "Lbp [m]"; Whead "Whead [m]"; Lhead "Lhead [m]"; Rhp "Rhp [m]"; Lhp "Lhp [m]"; circlePoints "Circle Mesh Resolution"; cylColor "Cylinder Color"; rhoCyl "Cylinder Density [kg/m^3]"; pistColor "Piston Color"; rhoPist "Piston Density [kg/m^3]"; connColor "Connector Color"; rhoConn "Connector Density [kg/m^3]"
      mask help:
      | Consists of the backhoe hydraulic actuator assembly.
      |
      | Zero piston displacement corresponds to the piston and cylinder centers of mass in the same position. Positive piston displacement is outward motion, and negative piston displacement is inward motion.
      |
      | Attachment points are:
      | C: Center of the Cylinder base bracket hole.
      | H: Center of the Piston Head bracket hole.
      | Both attachment points are configured for Revolute joints.
      |
      | The Simulink Signal input port supplies a Pressure value P (in Pa) to a Simscape hydraulic network.
      |
      | Click on Help to view a schematic of the hydraulic actuator, its configurable dimension parameters and attachment points (in red).
      mask init:
      | % Hollow Cylinder cross-section
      | cylSection = [];
      | 
      | for i = 0:2*circlePoints
      |     angle = (i/circlePoints)*pi;
      |     cylSection = [cylSection; Rcyl*cos(angle) Rcyl*sin(angle)];
      | end
      | 
      | for i = 0:2*circlePoints
      |     angle = -(i/circlePoints)*pi;
      |     cylSection = [cylSection; Rpist*cos(angle) Rpist*sin(angle)];
      | end
      mask Help: web(fullfile(matlabroot,'toolbox','physmod','sm','smdemos','backhoe','html','sm_backhoe_actuator.html'));
      mask Display:
      | image(imread('Backhoe_Arm_Actuator_IMAGE.jpg'));
      | port_label('lconn',1,'R');
      | port_label('lconn',2,'C');
      | port_label('rconn',1,'Cr');
      | port_label('rconn',2,'UA');
      | %port_label('input',1,'Cmd');
  UArm to Bucket : sm_lib/Joints/Revolute Joint  SenseConstraintForce=off  SenseConstraintForceX=off  SenseConstraintForceY=off  SenseConstraintForceZ=off  SenseConstraintTorque=off  SenseConstraintTorqueX=off  SenseConstraintTorqueY=off  SenseConstraintTorqueZ=off  SenseTotalForce=off  SenseTotalForceX=off  SenseTotalForceY=off  SenseTotalForceZ=off  SenseTotalTorque=off  SenseTotalTorqueX=off  SenseTotalTorqueY=off  SenseTotalTorqueZ=off  CompositeWrenchDir=FollowerOnBase  CompositeWrenchFrame=BaseFrame  EquilibriumPosition=0  EquilibriumPositionUnits=deg  SpringStiffness=0  SpringStiffnessUnits=N*m/deg  DampingCoefficient=0  DampingCoefficientUnits=N*m/(deg/s)  TorqueActuationMode=NoTorque  MotionActuationMode=ComputedMotion  SensePosition=on  SenseVelocity=off  SenseAcceleration=off  SenseTorqueForce=off  PositionTargetSpecify=on  PositionTargetPriority=High  PositionTargetValue=0  PositionTargetValueUnits=deg  VelocityTargetSpecify=off  VelocityTargetPriority=High  VelocityTargetValue=0  VelocityTargetValueUnits=deg/s
  UArm to CrankL : sm_lib/Joints/Revolute Joint  SenseConstraintForce=off  SenseConstraintForceX=off  SenseConstraintForceY=off  SenseConstraintForceZ=off  SenseConstraintTorque=off  SenseConstraintTorqueX=off  SenseConstraintTorqueY=off  SenseConstraintTorqueZ=off  SenseTotalForce=off  SenseTotalForceX=off  SenseTotalForceY=off  SenseTotalForceZ=off  SenseTotalTorque=off  SenseTotalTorqueX=off  SenseTotalTorqueY=off  SenseTotalTorqueZ=off  CompositeWrenchDir=FollowerOnBase  CompositeWrenchFrame=BaseFrame  EquilibriumPosition=0  EquilibriumPositionUnits=deg  SpringStiffness=0  SpringStiffnessUnits=N*m/deg  DampingCoefficient=0  DampingCoefficientUnits=N*m/(deg/s)  TorqueActuationMode=NoTorque  MotionActuationMode=ComputedMotion  SensePosition=off  SenseVelocity=off  SenseAcceleration=off  SenseTorqueForce=off  PositionTargetSpecify=off  PositionTargetPriority=Low  PositionTargetValue=-150  PositionTargetValueUnits=deg  VelocityTargetSpecify=off  VelocityTargetPriority=High  VelocityTargetValue=0  VelocityTargetValueUnits=deg/s
  UArm to CrankR : sm_lib/Joints/Revolute Joint  SenseConstraintForce=off  SenseConstraintForceX=off  SenseConstraintForceY=off  SenseConstraintForceZ=off  SenseConstraintTorque=off  SenseConstraintTorqueX=off  SenseConstraintTorqueY=off  SenseConstraintTorqueZ=off  SenseTotalForce=off  SenseTotalForceX=off  SenseTotalForceY=off  SenseTotalForceZ=off  SenseTotalTorque=off  SenseTotalTorqueX=off  SenseTotalTorqueY=off  SenseTotalTorqueZ=off  CompositeWrenchDir=FollowerOnBase  CompositeWrenchFrame=BaseFrame  EquilibriumPosition=0  EquilibriumPositionUnits=deg  SpringStiffness=0  SpringStiffnessUnits=N*m/deg  DampingCoefficient=0  DampingCoefficientUnits=N*m/(deg/s)  TorqueActuationMode=NoTorque  MotionActuationMode=ComputedMotion  SensePosition=off  SenseVelocity=off  SenseAcceleration=off  SenseTorqueForce=off  PositionTargetSpecify=off  PositionTargetPriority=High  PositionTargetValue=0  PositionTargetValueUnits=deg  VelocityTargetSpecify=off  VelocityTargetPriority=High  VelocityTargetValue=0  VelocityTargetValueUnits=deg/s
  UArm to TActuator : sm_lib/Joints/Revolute Joint  SenseConstraintForce=off  SenseConstraintForceX=off  SenseConstraintForceY=off  SenseConstraintForceZ=off  SenseConstraintTorque=off  SenseConstraintTorqueX=off  SenseConstraintTorqueY=off  SenseConstraintTorqueZ=off  SenseTotalForce=off  SenseTotalForceX=off  SenseTotalForceY=off  SenseTotalForceZ=off  SenseTotalTorque=off  SenseTotalTorqueX=off  SenseTotalTorqueY=off  SenseTotalTorqueZ=off  CompositeWrenchDir=FollowerOnBase  CompositeWrenchFrame=BaseFrame  EquilibriumPosition=0  EquilibriumPositionUnits=deg  SpringStiffness=0  SpringStiffnessUnits=N*m/deg  DampingCoefficient=0  DampingCoefficientUnits=N*m/(deg/s)  TorqueActuationMode=NoTorque  MotionActuationMode=ComputedMotion  SensePosition=off  SenseVelocity=off  SenseAcceleration=off  SenseTorqueForce=off  PositionTargetSpecify=on  PositionTargetPriority=Low  PositionTargetValue=-90  PositionTargetValueUnits=deg  VelocityTargetSpecify=off  VelocityTargetPriority=High  VelocityTargetValue=0  VelocityTargetValueUnits=deg/s
  Upper Arm : Subsystem
      mask Display:
      | image(imread('Backhoe_Arm_Upper_IMAGE.JPG'));
      | port_label('lconn',1,'LA');
      | port_label('lconn',2,'RAct');
      | port_label('rconn',1,'CrL');
      | port_label('rconn',2,'CrR');
      | port_label('rconn',3,'B');
      | port_label('rconn',4,'TAct');
  World Frame : sm_lib/Frames and Transforms/World Frame
  C : PMIOPort  Side=Left
  R : PMIOPort  Port=2  Side=Left
  B : Outport
  wires:
  [BuA] -> B/1
  connections:
  Friction/LConn1 -- Sensing/RConn1 -- Tilt Actuator/LConn1
  World Frame/RConn1 -- Upper Arm/LConn1 -- Solver Config/RConn1 -- Mech Config/RConn1
  Upper Arm/RConn3 -- UArm to Bucket/LConn1
  Bucket Assembly/LConn3 -- UArm to Bucket/RConn1
  UArm to TActuator/RConn1 -- Tilt Actuator/RConn2
  Bucket Assembly/RConn1 -- Tilt Actuator/RConn1
  Bucket Assembly/LConn2 -- UArm to CrankR/RConn1
  Upper Arm/RConn2 -- UArm to CrankR/LConn1
  Upper Arm/RConn4 -- UArm to TActuator/LConn1
  Upper Arm/RConn1 -- UArm to CrankL/LConn1
  Sensing AB/LConn1 -- UArm to Bucket/RConn2
  Bucket Assembly/LConn1 -- UArm to CrankL/RConn1
  Friction/RConn1 -- C/RConn1 -- Tilt Actuator/LConn2
  Sensing/LConn1 -- R/RConn1

== system Backhoe_TiltCyl_PIopt/Units ==
  S : Inport
  Convert Valve Disp : Gain  Gain=1e-5
  Simulink-PS Converter : nesl_utility/Simulink-PS Converter  PhysicalDomain=network_engine_domain  SubClassName=ps_input  LeftPortType=input  RightPortType=output  PseudoPeriodic=off  Frequencies=[]  NoiseDistribution=none  NoiseParameters=[]  Unit=m  AffineConversion=off  FilteringAndDerivatives=provide  SimscapeFilterOrder=1  InputFilterTimeConstant=.001  UdotUserProvided=0
  PS : PMIOPort  Side=Right
  wires:
  S/1 -> Convert Valve Disp/1
  Convert Valve Disp/1 -> Simulink-PS Converter/1
  connections:
  Simulink-PS Converter/RConn1 -- PS/RConn1

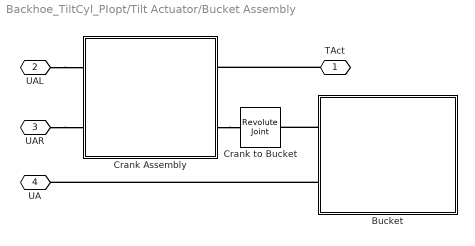
== system Backhoe_TiltCyl_PIopt/Tilt Actuator/Bucket Assembly ==
  Bucket : Subsystem  mask(Bucket){plateSide=1.2, plateFilletR=0.2, plateDist=1.2, plateWidth=0.2, plateHoleR=0.075, bucketHeight=2, bucketLength=2, bucketThickness=0.05, bucketUpper=1.3, bucketLower=2, chordAngle=pi/6, toothLength=0.25, toothWidth=0.2, toothTip=0.025, circlePoints=45, bucketColor=yellow, bracketColor=yellow, rho=rhoSteel}
      mask prompts: plateSide "Wplate [m]"; plateFilletR "Rfillet [m]"; plateDist "Dplate [m]"; plateWidth "Tplate [m]"; plateHoleR "Rpin [m]"; bucketHeight "Hbucket [m]"; bucketLength "Wbucket [m]"; bucketThickness "Tbucket [m]"; bucketUpper "Wupper [m]"; bucketLower "Wlower [m]"; chordAngle "alpha [radians]"; toothLength "Ltooth [m]"; toothWidth "Wtooth [m]"; toothTip "Ttooth [m]"; circlePoints "Circle Mesh Resolution"; bucketColor "Bucket Color"; bracketColor "Bracket Color"; rho "Density [kg/m^3]"
      mask help:
      | Consists of the backhoe bucket assembly with attachment frame.
      |
      | Attachment points are:
      | CA: Center point of the Crank Arm link pin.
      | UA: Center Point of the Upper Arm link pin.
      | Both points are configured for Revolute joints.
      |
      | Click on Help to view a schematic of the bucket, its configurable dimension parameters and attachment points (in red).
      mask init:
      | bucketRadius = bucketHeight/(2*cos(chordAngle));
      | 
      | % Bucket Back
      | bucketBack = [];
      | % Outer wall
      | for i = 0:circlePoints;
      |    angle = (-pi/2+chordAngle) + (pi - 2*chordAngle)*(i/circlePoints);
      |    bucketBack = [bucketBack; ...
      |        (bucketRadius*cos(angle)-bucketRadius*sin(chordAngle)) ...
      |         bucketRadius*sin(angle)];
      | end
      | 
      | % Inner Wall
      | beta = acos( ( (bucketRadius*cos(chordAngle) - bucketThickness/cos(chordAngle)) ...
      |                    /(bucketRadius-bucketThickness)) );
      | for i = 0:circlePoints;
      |    angle = (pi/2 - beta) - (pi-2*beta)*(i/circlePoints);
      |    bucketBack = [bucketBack; ...
      |        ((bucketRadius-bucketThickness)*cos(angle)-bucketRadius*sin(chordAngle)) ... 
      |        (bucketRadius-bucketThickness)*sin(angle)];
      | end
      | 
      | bucketBack = [bucketBack; ...
      |               -bucketLower -(bucketHeight/2-bucketThickness);...
      |               -bucketLower -bucketHeight/2];
      |           
      | % Uncomment below to plot the cross-sections. 
      | % close all
      | % figure
      | % plot(bucketBack(:,1),bucketBack(:,2));
      mask Help: web('Backhoe_Bucket.html');
      mask Display:
      | image(imread('Backhoe_Bucket_IMAGE.png'));
      | port_label('rconn',1,'CA');
      | port_label('rconn',2,'UA');
  Crank Assembly : Subsystem  mask(Crank Assembly){LC1=1.5, WC1=0.4, TC1=0.2, DH1=1.1, RH1=0.075, LC2=1.75, WC2=0.4, TC2=0.15, DH2=1.35, RH2=0.075, DC2=0.7, Wbar=0.8, Lpin=1.3, Rpin=0.075, circlePoints=25, color1=orange, color2=darkOrange, rho1=rhoSteel, rho2=rhoSteel}
      mask prompts: LC1 "LC1 [m]"; WC1 "WC1 [m]"; TC1 "TC1 [m]"; DH1 "DH1 [m]"; RH1 "RH1 [m]"; LC2 "LC2 [m]"; WC2 "WC2 [m]"; TC2 "TC2 [m]"; DH2 "DH2 [m]"; RH2 "RH2 [m]"; DC2 "DC2 [m]"; Wbar "Upper Arm Width, Wbar [m]"; Lpin "Lpin [m]"; Rpin "Rpin [m]"; circlePoints "Circle Mesh Resolution"; color1 "Color"; color2 "Color"; rho1 "Density [kg/m^3]"; rho2 "Density [kg/m^3]"
      mask help:
      | Consists of the backhoe crank assembly that connects the upper arm and the bucket. Crank 1 attaches to either side of the upper arm linkage, and Crank 2 connects Crank 1 and the Bucket.
      |
      | Attachment points are:
      | AL: Arm attachment (Left).
      | AR: Arm attachment (Right).
      | B: Bucket attachment.
      | P: Piston attachment.
      | All attachment points are configured for Revolute joints.
      |
      | Click on Help to view a schematic of the crank assembly, its configurable dimension parameters and attachment points (in red).
      mask Help: web('Backhoe_Crank.html');
      mask Display:
      | image(imread('Backhoe_Crankassembly_IMAGE.png'));
      | port_label('rconn',1,'B');
      | port_label('rconn',2,'P');
      | port_label('lconn',1,'AL');
      | port_label('lconn',2,'AR');
  Crank to Bucket : sm_lib/Joints/Revolute Joint  SenseConstraintForce=off  SenseConstraintForceX=off  SenseConstraintForceY=off  SenseConstraintForceZ=off  SenseConstraintTorque=off  SenseConstraintTorqueX=off  SenseConstraintTorqueY=off  SenseConstraintTorqueZ=off  SenseTotalForce=off  SenseTotalForceX=off  SenseTotalForceY=off  SenseTotalForceZ=off  SenseTotalTorque=off  SenseTotalTorqueX=off  SenseTotalTorqueY=off  SenseTotalTorqueZ=off  CompositeWrenchDir=FollowerOnBase  CompositeWrenchFrame=BaseFrame  EquilibriumPosition=0  EquilibriumPositionUnits=deg  SpringStiffness=0  SpringStiffnessUnits=N*m/deg  DampingCoefficient=0  DampingCoefficientUnits=N*m/(deg/s)  TorqueActuationMode=NoTorque  MotionActuationMode=ComputedMotion  SensePosition=off  SenseVelocity=off  SenseAcceleration=off  SenseTorqueForce=off  PositionTargetSpecify=off  PositionTargetPriority=Low  PositionTargetValue=0  PositionTargetValueUnits=deg  VelocityTargetSpecify=off  VelocityTargetPriority=High  VelocityTargetValue=0  VelocityTargetValueUnits=deg/s
  TAct : PMIOPort  Side=Right
  UAL : PMIOPort  Port=2  Side=Left
  UAR : PMIOPort  Port=3  Side=Left
  UA : PMIOPort  Port=4  Side=Left
  connections:
  Bucket/RConn1 -- Crank to Bucket/RConn1
  Crank Assembly/RConn2 -- Crank to Bucket/LConn1
  Bucket/RConn2 -- UA/RConn1
  UAL/RConn1 -- Crank Assembly/LConn1
  UAR/RConn1 -- Crank Assembly/LConn2
  TAct/RConn1 -- Crank Assembly/RConn1

== system Backhoe_TiltCyl_PIopt/Tilt Actuator/Sensing ==
  Ideal Force Sensor : fl_lib/Mechanical/Mechanical Sensors/Ideal Force Sensor
  PS-Simulink Converter : nesl_utility/PS-Simulink Converter  PhysicalDomain=network_engine_domain  SubClassName=ps_output  LeftPortType=input  RightPortType=output  PseudoPeriodic=off  Frequencies=[]  Unit=1  AffineConversion=off
  C : PMIOPort  Side=Right
  R : PMIOPort  Port=2  Side=Left
  tag scope: Tilt_Act_F=global
  wires:
  PS-Simulink Converter/1 -> [Tilt_Act_F]
  connections:
  Ideal Force Sensor/LConn1 -- R/RConn1
  Ideal Force Sensor/RConn1 -- C/RConn1
  PS-Simulink Converter/LConn1 -- Ideal Force Sensor/RConn2

== system Backhoe_TiltCyl_PIopt/Tilt Actuator/Sensing AB ==
  PS-Simulink Converter Upper1 : nesl_utility/PS-Simulink Converter  PhysicalDomain=network_engine_domain  SubClassName=ps_output  LeftPortType=input  RightPortType=output  PseudoPeriodic=off  Frequencies=[]  Unit=deg  AffineConversion=off
  Conn1 : PMIOPort  Side=Left
  tag scope: BuA=global
  wires:
  PS-Simulink Converter Upper1/1 -> [BuA]
  connections:
  PS-Simulink Converter Upper1/LConn1 -- Conn1/RConn1

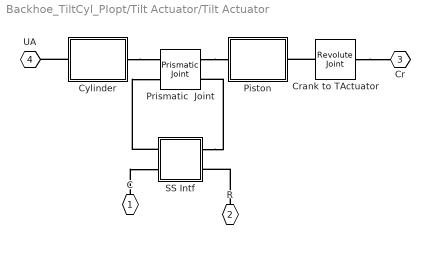
== system Backhoe_TiltCyl_PIopt/Tilt Actuator/Tilt Actuator ==
  Crank to TActuator : sm_lib/Joints/Revolute Joint  SenseConstraintForce=off  SenseConstraintForceX=off  SenseConstraintForceY=off  SenseConstraintForceZ=off  SenseConstraintTorque=off  SenseConstraintTorqueX=off  SenseConstraintTorqueY=off  SenseConstraintTorqueZ=off  SenseTotalForce=off  SenseTotalForceX=off  SenseTotalForceY=off  SenseTotalForceZ=off  SenseTotalTorque=off  SenseTotalTorqueX=off  SenseTotalTorqueY=off  SenseTotalTorqueZ=off  CompositeWrenchDir=FollowerOnBase  CompositeWrenchFrame=BaseFrame  EquilibriumPosition=0  EquilibriumPositionUnits=deg  SpringStiffness=0  SpringStiffnessUnits=N*m/deg  DampingCoefficient=0  DampingCoefficientUnits=N*m/(deg/s)  TorqueActuationMode=NoTorque  MotionActuationMode=ComputedMotion  SensePosition=off  SenseVelocity=off  SenseAcceleration=off  SenseTorqueForce=off  PositionTargetSpecify=off  PositionTargetPriority=High  PositionTargetValue=0  PositionTargetValueUnits=deg  VelocityTargetSpecify=off  VelocityTargetPriority=High  VelocityTargetValue=0  VelocityTargetValueUnits=deg/s
  Cylinder : Subsystem
  Piston : Subsystem
  Prismatic  Joint : sm_lib/Joints/Prismatic Joint  SenseConstraintForce=off  SenseConstraintForceX=off  SenseConstraintForceY=off  SenseConstraintForceZ=off  SenseConstraintTorque=off  SenseConstraintTorqueX=off  SenseConstraintTorqueY=off  SenseConstraintTorqueZ=off  SenseTotalForce=off  SenseTotalForceX=off  SenseTotalForceY=off  SenseTotalForceZ=off  SenseTotalTorque=off  SenseTotalTorqueX=off  SenseTotalTorqueY=off  SenseTotalTorqueZ=off  CompositeWrenchDir=FollowerOnBase  CompositeWrenchFrame=BaseFrame  EquilibriumPosition=0  EquilibriumPositionUnits=m  SpringStiffness=0  SpringStiffnessUnits=N/m  DampingCoefficient=0  DampingCoefficientUnits=N/(m/s)  TorqueActuationMode=InputTorque  MotionActuationMode=ComputedMotion  SensePosition=off  SenseVelocity=on  SenseAcceleration=off  SenseTorqueForce=off  PositionTargetSpecify=off  PositionTargetPriority=Low  PositionTargetValue=0  PositionTargetValueUnits=m  VelocityTargetSpecify=off  VelocityTargetPriority=High  VelocityTargetValue=0  VelocityTargetValueUnits=m/s
  SS Intf : Subsystem
  C : PMIOPort  Side=Left
  R : PMIOPort  Port=2  Side=Left
  Cr : PMIOPort  Port=3  Side=Right
  UA : PMIOPort  Port=4  Side=Right
  connections:
  R/RConn1 -- SS Intf/LConn2
  C/RConn1 -- SS Intf/RConn2
  SS Intf/RConn1 -- Prismatic  Joint/LConn2
  SS Intf/LConn1 -- Prismatic  Joint/RConn2
  Prismatic  Joint/RConn1 -- Piston/LConn1
  Cylinder/LConn1 -- Prismatic  Joint/LConn1
  Crank to TActuator/LConn1 -- Piston/RConn1
  Crank to TActuator/RConn1 -- Cr/RConn1
  Cylinder/RConn1 -- UA/RConn1

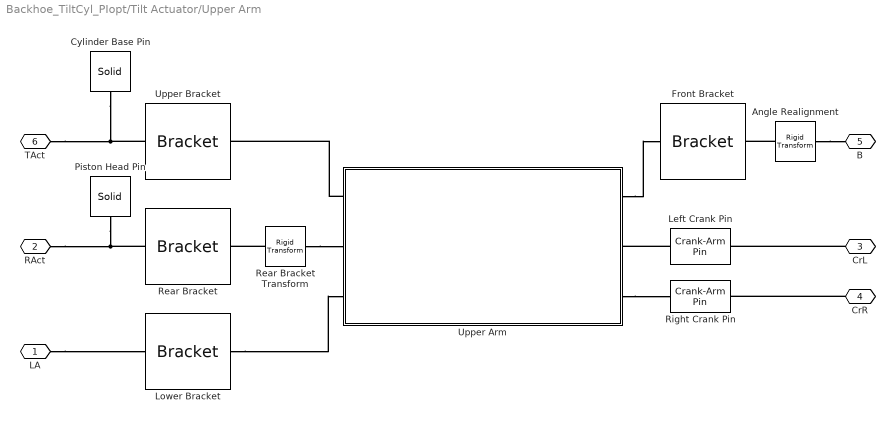
== system Backhoe_TiltCyl_PIopt/Tilt Actuator/Upper Arm ==
  Angle Realignment : sm_lib/Frames and Transforms/Rigid Transform  TranslationMethod=None  TranslationStandardOffset=0  TranslationLengthUnit=m  TranslationStandardAxis=+Z  TranslationCartesianOffset=[0 0 0]  TranslationROffset=0  TranslationROffsetUnits=m  TranslationZOffset=0  TranslationZOffsetUnits=m  TranslationThetaOffset=0  TranslationThetaOffsetUnits=deg  RotationMethod=AlignedAxes  RotationAngleUnits=deg  RotationStandardAxis=-Z  RotationAngle=90  RotationArbitraryAxis=[0 0 1]  FollAlignAxisA=+X  BaseAlignAxisA=-Y  FollAlignAxisB=+Z  BaseAlignAxisB=+Z  RotationSequenceAxes=FollowerAxes  RotationSequence=XYX  RotationSequenceAngles=[0 0 0]  RotationSequenceAnglesUnits=deg  RotationMatrix=[1 0 0; 0 1 0; 0 0 1]
  Cylinder Base Pin : sm_lib/Body Elements/Solid  InertiaType=CalculateFromGeometry  Mass=1  MassUnits=kg  CenterOfMass=[0 0 0]  CenterOfMassUnits=m  MomentsOfInertia=[1 1 1]  MomentsOfInertiaUnits=kg*m^2  ProductsOfInertia=[0 0 0]  ProductsOfInertiaUnits=kg*m^2  DensityBased=on  Density=rhoSteel  DensityUnits=kg/(m^3)  DoExposeReferenceFrame=on  SerializedFrames=<Frames/>  GraphicType=FromGeometry  MarkerShape=Sphere  MarkerSize=10  MarkerSizeUnits=m  GraphicVisPropType=SimpleVisualProperties  GraphicDiffuseColor=gray  GraphicSpecularColor=[0.5 0.5 0.5 1.0]  GraphicAmbientColor=[0.15 0.15 0.15 1.0]  GraphicEmissiveColor=[0.0 0.0 0.0 1.0]  GraphicShininess=75  GraphicOpacity=1.0  GeometryShape=Cylinder  RectangleSize=[1 1]  RectangleSizeUnits=m  BrickDimensions=[3 0.5 0.5]  BrickDimensionUnits=m  CylinderRadius=0.075  CylinderRadiusUnits=m  CylinderLength=0.8  CylinderLengthUnits=m  SphereRadius=1  SphereRadiusUnits=m  EllipsoidRadii=[1 1 1]  EllipsoidRadiiUnits=m  ExtrusionCrossSection=[1 1; -1 1; -1 -1; 1 -1]  ExtrusionCrossSectionUnits=m  ExtrusionLength=1  ExtrusionLengthUnits=m  PolygonNumSides=3  PolygonOuterRadius=1  PolygonOuterRadiusUnits=m  ExtGeomFileType=STL  ExtGeomFileUnits=m  RevolutionCrossSection=[1 1; 1 -1; 2 -1; 2 1]  RevolutionCrossSectionUnits=m  RevolutionExtent=Full  RevolutionAngle=180  RevolutionAngleUnits=deg
  Front Bracket : Backhoe_Lib/Bracket  Hbracket=0.65  Wbracket=0.5  Tbracket=0.15  Dbracket=0.625  Hhole=0.4  Rhole=0.075  circlePoints=25  bracketColor=orange  rho=rhoSteel
  Left Crank Pin : Backhoe_Lib/Crank-Arm Pin  R=0.075  L=0.25  T=0.2  color=gray  rho=rhoSteel
  Lower Bracket : Backhoe_Lib/Bracket  Hbracket=0.75  Wbracket=0.75  Tbracket=0.15  Dbracket=0.75  Hhole=0.5  Rhole=0.075  circlePoints=25  bracketColor=orange  rho=rhoSteel
  Piston Head Pin : sm_lib/Body Elements/Solid  InertiaType=CalculateFromGeometry  Mass=1  MassUnits=kg  CenterOfMass=[0 0 0]  CenterOfMassUnits=m  MomentsOfInertia=[1 1 1]  MomentsOfInertiaUnits=kg*m^2  ProductsOfInertia=[0 0 0]  ProductsOfInertiaUnits=kg*m^2  DensityBased=on  Density=rhoSteel  DensityUnits=kg/(m^3)  DoExposeReferenceFrame=on  SerializedFrames=<Frames/>  GraphicType=FromGeometry  MarkerShape=Sphere  MarkerSize=10  MarkerSizeUnits=m  GraphicVisPropType=SimpleVisualProperties  GraphicDiffuseColor=gray  GraphicSpecularColor=[0.5 0.5 0.5 1.0]  GraphicAmbientColor=[0.15 0.15 0.15 1.0]  GraphicEmissiveColor=[0.0 0.0 0.0 1.0]  GraphicShininess=75  GraphicOpacity=1.0  GeometryShape=Cylinder  RectangleSize=[1 1]  RectangleSizeUnits=m  BrickDimensions=[1 1 1]  BrickDimensionUnits=m  CylinderRadius=0.075  CylinderRadiusUnits=m  CylinderLength=0.8  CylinderLengthUnits=m  SphereRadius=1  SphereRadiusUnits=m  EllipsoidRadii=[1 1 1]  EllipsoidRadiiUnits=m  ExtrusionCrossSection=[1 1; -1 1; -1 -1; 1 -1]  ExtrusionCrossSectionUnits=m  ExtrusionLength=1  ExtrusionLengthUnits=m  PolygonNumSides=3  PolygonOuterRadius=1  PolygonOuterRadiusUnits=m  ExtGeomFileType=STL  ExtGeomFileUnits=m  RevolutionCrossSection=[1 1; 1 -1; 2 -1; 2 1]  RevolutionCrossSectionUnits=m  RevolutionExtent=Full  RevolutionAngle=180  RevolutionAngleUnits=deg
  Rear Bracket : Backhoe_Lib/Bracket  Hbracket=0.75  Wbracket=0.75  Tbracket=0.15  Dbracket=0.75  Hhole=0.5  Rhole=0.075  circlePoints=25  bracketColor=orange  rho=rhoSteel
  Rear Bracket Transform : sm_lib/Frames and Transforms/Rigid Transform  TranslationMethod=None  TranslationStandardOffset=0.5  TranslationLengthUnit=m  TranslationStandardAxis=+Z  TranslationCartesianOffset=[ 0 0 0]  TranslationROffset=0  TranslationROffsetUnits=m  TranslationZOffset=0  TranslationZOffsetUnits=m  TranslationThetaOffset=0  TranslationThetaOffsetUnits=deg  RotationMethod=AlignedAxes  RotationAngleUnits=deg  RotationStandardAxis=+X  RotationAngle=90  RotationArbitraryAxis=[0 0 1]  FollAlignAxisA=+Z  BaseAlignAxisA=+Z  FollAlignAxisB=+Y  BaseAlignAxisB=-Y  RotationSequenceAxes=FollowerAxes  RotationSequence=XYX  RotationSequenceAngles=[0 0 0]  RotationSequenceAnglesUnits=deg  RotationMatrix=[1 0 0; 0 1 0; 0 0 1]
  Right Crank Pin : Backhoe_Lib/Crank-Arm Pin  R=0.075  L=0.25  T=0.2  color=gray  rho=rhoSteel
  Upper Arm : Subsystem  mask(Upper Arm){Lbar=6, Wbar=0.8, Tbar=0.85, L1=1.5, L2=1.5, L3=2.5, barFillet=0.1, numPoints=15, Tcrank=0.2, armColor=yellow, rho=rhoSteel}
      mask prompts: Lbar "Lbar [m]"; Wbar "Wbar [m]"; Tbar "Tbar [m]"; L1 "L1 [m]"; L2 "L2 [m]"; L3 "L3 [m]"; barFillet "Bar Fillet Radius [m]"; numPoints "Fillet Point Resolution"; Tcrank "Crank Arm Thickness [m]"; armColor "Arm Color"; rho "Density [kg/m^3]"
      mask help:
      | Consists of the backhoe upper arm and four attachment brackets -- front, rear, upper and lower.
      |
      | Attachment points are:
      | B: Bucket attachment.
      | CL: Crank arm attachment (Left).
      | CR: Crank arm attachment (Right).
      | BC: Bucket hydraulic actuator (Cylinder base).
      | LA: Lower Arm attachment.
      | UH: Upper arm hydraulic actuator (piston Head).
      | All attachment points are configured for Revolute joints.
      |
      | The lengths L1, L2 and L3 correspond to lengths measured from the center of the bar, as follows:
      | L1: Upper Bracket
      | L2: Lower Bracket
      | L3: Crank Attachment Points
      | The front and rear brackets are automatically placed at the center of the end faces of the upper arm bar.
      |
      | Click on Help to view a schematic of the upper arm, its configurable dimension parameters and attachment points (in red).
      mask init:
      | barSection = [Tbar/2 Wbar/2;  ...
      |              -Tbar/2 Wbar/2;  ...
      |              -Tbar/2 -Wbar/2; ...
      |               Tbar/2 -Wbar/2];
      | barSection = Extr_Data_Round_Corners(barSection,1:4,barFillet,numPoints);
      mask Help: web('Backhoe_Upperarm.html');
      mask Display:
      | image(imread('Backhoe_Upperbar_IMAGE.png'));
      | port_label('lconn',1,'CB');
      | port_label('lconn',2,'PH');
      | port_label('lconn',3,'LA');
      | port_label('rconn',1,'B');
      | port_label('rconn',2,'CL');
      | port_label('rconn',3,'CR');
  Upper Bracket : Backhoe_Lib/Bracket  Hbracket=0.75  Wbracket=0.75  Tbracket=0.15  Dbracket=0.75  Hhole=0.5  Rhole=0.075  circlePoints=25  bracketColor=orange  rho=rhoSteel
  LA : PMIOPort  Side=Left
  RAct : PMIOPort  Port=2  Side=Left
  CrL : PMIOPort  Port=3  Side=Right
  CrR : PMIOPort  Port=4  Side=Right
  B : PMIOPort  Port=5  Side=Right
  TAct : PMIOPort  Port=6  Side=Right
  connections:
  Cylinder Base Pin/RConn1 -- Upper Bracket/RConn1 -- TAct/RConn1
  Piston Head Pin/RConn1 -- RAct/RConn1 -- Rear Bracket/RConn1
  Angle Realignment/LConn1 -- Front Bracket/RConn1
  LA/RConn1 -- Lower Bracket/RConn1
  CrL/RConn1 -- Left Crank Pin/LConn1
  CrR/RConn1 -- Right Crank Pin/LConn1
  Rear Bracket Transform/RConn1 -- Rear Bracket/LConn1
  Upper Arm/LConn1 -- Upper Bracket/LConn1
  Upper Arm/RConn1 -- Front Bracket/LConn1
  Upper Arm/RConn3 -- Right Crank Pin/RConn1
  Lower Bracket/LConn1 -- Upper Arm/LConn3
  Rear Bracket Transform/LConn1 -- Upper Arm/LConn2
  Left Crank Pin/RConn1 -- Upper Arm/RConn2
  Angle Realignment/RConn1 -- B/RConn1

== system Backhoe_TiltCyl_PIopt/Tilt Actuator/Bucket Assembly/Bucket ==
  Arm Revolute Rotation : sm_lib/Frames and Transforms/Rigid Transform  TranslationMethod=None  TranslationStandardOffset=0  TranslationLengthUnit=m  TranslationStandardAxis=+X  TranslationCartesianOffset=[0 0 0]  TranslationROffset=0  TranslationROffsetUnits=m  TranslationZOffset=0  TranslationZOffsetUnits=m  TranslationThetaOffset=0  TranslationThetaOffsetUnits=deg  RotationMethod=AlignedAxes  RotationAngleUnits=deg  RotationStandardAxis=-Y  RotationAngle=180  RotationArbitraryAxis=[0 0 1]  FollAlignAxisA=+Y  BaseAlignAxisA=+Y  FollAlignAxisB=+X  BaseAlignAxisB=-X  RotationSequenceAxes=FollowerAxes  RotationSequence=XYX  RotationSequenceAngles=[0 0 0]  RotationSequenceAnglesUnits=deg  RotationMatrix=[1 0 0; 0 1 0; 0 0 1]
  Attachment Frame : Subsystem
      mask Display:
      | image(imread('Backhoe_Attach_IMAGE.png'));
      | port_label('lconn',1,'B');
      | port_label('rconn',1,'CA');
      | port_label('rconn',2,'UA');
  Bucket : Subsystem
      mask Display:
      | image(imread('Backhoe_Bucketcase_IMAGE.png'));
      | port_label('rconn',1,'AF');
  Crank Revolute Rotation : sm_lib/Frames and Transforms/Rigid Transform  TranslationMethod=None  TranslationStandardOffset=0  TranslationLengthUnit=m  TranslationStandardAxis=+X  TranslationCartesianOffset=[0 0 0]  TranslationROffset=0  TranslationROffsetUnits=m  TranslationZOffset=0  TranslationZOffsetUnits=m  TranslationThetaOffset=0  TranslationThetaOffsetUnits=deg  RotationMethod=AlignedAxes  RotationAngleUnits=deg  RotationStandardAxis=-Y  RotationAngle=180  RotationArbitraryAxis=[0 0 1]  FollAlignAxisA=+Y  BaseAlignAxisA=+Y  FollAlignAxisB=+X  BaseAlignAxisB=-X  RotationSequenceAxes=FollowerAxes  RotationSequence=XYX  RotationSequenceAngles=[0 0 0]  RotationSequenceAnglesUnits=deg  RotationMatrix=[1 0 0; 0 1 0; 0 0 1]
  Crank Arm : PMIOPort  Side=Right
  Upper Arm : PMIOPort  Port=2  Side=Right
  connections:
  Bucket/RConn1 -- Attachment Frame/LConn1
  Crank Revolute Rotation/LConn1 -- Attachment Frame/RConn1
  Arm Revolute Rotation/LConn1 -- Attachment Frame/RConn2
  Upper Arm/RConn1 -- Arm Revolute Rotation/RConn1
  Crank Arm/RConn1 -- Crank Revolute Rotation/RConn1
